simulink model "PV_MPPT"  (R2022b)
settings: Solver=VariableStepAuto  StartTime=0.0  StopTime=0.2  RelTol=1e-3
model workspace (MAT data in the model file):
  Tn = 298
undefined symbols (not defined in the file): sigbuilder_block
libraries: spsSeriesRLCBranchLib x4, spsCurrentMeasurementLib x1, spsGroundLib x1, spsIGBTLib x1, spsControlledCurrentSourceLib x1, spsPWMGeneratorDCDCLib x1, simulink x1, spsDiodeLib x1, spsVoltageMeasurementLib x1, spspowerguiLib x1
settings Model: Creator=Administrator  LastModifiedBy=58239
settings DebuggingCC: AlgebraicLoopMsg=none
settings ModelReferenceCC: EnableRefExpFcnMdlSchedulingChecks=on

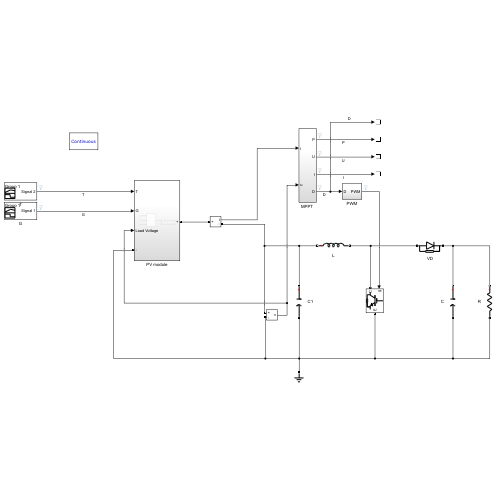
[thumbnail: Simulink's stored preview of the top-level diagram]
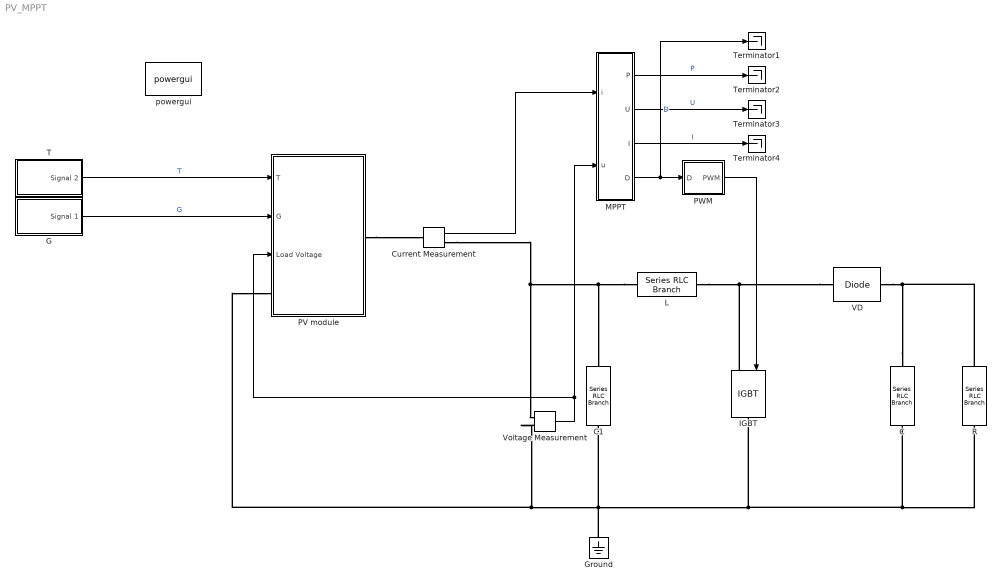
== system PV_MPPT ==
  C : spsSeriesRLCBranchLib/Series RLC Branch  LConnTagsString=__new0  RConnTagsString=__new0  BranchType=C  Resistance=0  Inductance=0  SetiL0=off  InitialCurrent=0  Capacitance=300e-6  Setx0=on  InitialVoltage=0  Measurements=None
  C1 : spsSeriesRLCBranchLib/Series RLC Branch  LConnTagsString=__new0  RConnTagsString=__new0  BranchType=C  Resistance=0  Inductance=0  SetiL0=off  InitialCurrent=0  Capacitance=300e-6  Setx0=off  InitialVoltage=0  Measurements=None
  Current Measurement : spsCurrentMeasurementLib/Current Measurement  PhasorSimulation=off  OutputType=Complex  PSBequivalent=0
  G : Subsystem  Tag=STV Subsys  LoadFcn=sigbuilder_block('load');  StartFcn=sigbuilder_block('start');  StopFcn=sigbuilder_block('stop');  ClipboardFcn=sigbuilder_block('clipboard');  mask(Sigbuilder block){tuvar=[0:10]}
      mask help: Sigbuilder GUI
      mask init:
      | if ~strcmp(get_param(bdroot(gcbh),'SimulationStatus'),'stopped') tuvar = sigbuilder_block('maskInit'); end
      settings: CopyFcn=sigbuilder_block('copy');  DeleteFcn=sigbuilder_block('delete');  ModelCloseFcn=sigbuilder_block('modelClose');  PreSaveFcn=sigbuilder_block('preSave');  PauseFcn=sigbuilder_block('pause')  ContinueFcn=sigbuilder_block('continue')  NameChangeFcn=sigbuilder_block('namechange');  OpenFcn=sigbuilder_block('open',[291 78 519 442.2 ]);  CloseFcn=sigbuilder_block('close');
      mask Display: plot(0, 0, 100, 100,[2, 2, 32, 32, 2], [68, 8, 8, 68, 68],[32, 2], [38, 38], [32, 19, 2],[53, 60, 44], [32, 17, 17, 2],[16, 16, 31, 31]);txt = getActiveGroup(gcbh);text(2, 100, txt,'verticalAlignment', 'top');
  Ground : spsGroundLib/Ground  LConnTagsString=a
  IGBT : spsIGBTLib/IGBT  Ron=0.00000001  Lon=0  Vf=1  Tf=1e-6  Tt=2e-6  IC=0  Rs=1e5  Cs=inf  Measurements=off
  L : spsSeriesRLCBranchLib/Series RLC Branch  LConnTagsString=__new0  RConnTagsString=__new0  BranchType=L  Resistance=0  Inductance=200e-6  SetiL0=off  InitialCurrent=1  Capacitance=inf  Setx0=off  InitialVoltage=0  Measurements=None
  "MPPT " : Subsystem
  PV module : Subsystem
  PWM : Subsystem
  R : spsSeriesRLCBranchLib/Series RLC Branch  LConnTagsString=__new0  RConnTagsString=__new0  BranchType=R  Resistance=30  Inductance=100e-6  SetiL0=off  InitialCurrent=0  Capacitance=inf  Setx0=off  InitialVoltage=0  Measurements=None
  T : Subsystem  Tag=STV Subsys  LoadFcn=sigbuilder_block('load');  StartFcn=sigbuilder_block('start');  StopFcn=sigbuilder_block('stop');  ClipboardFcn=sigbuilder_block('clipboard');  mask(Sigbuilder block){tuvar=[0:10]}
      mask help: Sigbuilder GUI
      mask init:
      | if ~strcmp(get_param(bdroot(gcbh),'SimulationStatus'),'stopped') tuvar = sigbuilder_block('maskInit'); end
      settings: CopyFcn=sigbuilder_block('copy');  DeleteFcn=sigbuilder_block('delete');  ModelCloseFcn=sigbuilder_block('modelClose');  PreSaveFcn=sigbuilder_block('preSave');  PauseFcn=sigbuilder_block('pause')  ContinueFcn=sigbuilder_block('continue')  NameChangeFcn=sigbuilder_block('namechange');  OpenFcn=sigbuilder_block('open',[317 199.5 519.5 400 ]);  CloseFcn=sigbuilder_block('close');
      mask Display: plot(0, 0, 100, 100,[2, 2, 32, 32, 2], [68, 8, 8, 68, 68],[32, 2], [38, 38], [32, 19, 2],[53, 60, 44], [32, 17, 17, 2],[16, 16, 31, 31]);txt = getActiveGroup(gcbh);text(2, 100, txt,'verticalAlignment', 'top');
  Terminator{1..4} (4 alike) : Terminator
  VD : spsDiodeLib/Diode  Ron=0.00000001  Lon=0  Vf=0.7  IC=0  UseSnubber=off  Rs=500  Cs=250e-9  Measurements=off
  Voltage Measurement : spsVoltageMeasurementLib/Voltage Measurement  PhasorSimulation=off  OutputType=Complex  PSBequivalent=0
  powergui : spspowerguiLib/powergui  Priority=1  SimulationMode=Continuous  SampleTime=50e-8  frequency=60  Iterations=50  frequencyindice=0  Pbase=100e6  ErrMax=1e-4  UnitsV=kV  UnitsW=MW  buscounter=0  FunctionMessages=off  echomessages=off  EnableUseOfTLC=off  CurrentSourceSwitches=off  DisableSnubberDevices=off  DisableRonSwitches=off  DisableVfSwitches=off  DisplayEquations=off  AutomaticDiscreteSolvers=off  SolverType=Tustin/Backward Euler (TBE)  Interpol=off  ExternalGateDelay=off  methode=off  Ts=100  x0status=blocks  SPID=off  SwTol=0  HookPort=off  NonlinearTolerance=1e-4  nMaxIteration=100  ContinueOnMaxIteration=off  RestoreLinks=warning  ResistiveCurrentMeasurement=off  Frange=[0:2:500]  Ylog=off  Xlog=on  ShowGrid=off  save=off  variable=ZData  structure=0  ZoomFFT=off  StartTime=0.0  cycles=1  DisplayStyle=1  fundamental=60  FreqAxis=off  MaxFrequency=1000  frequencyindicesteady=1  RmsSteady=1  display=off
  wires:
  "MPPT "/4(D) -> Terminator1/1, PWM/1(D)  "D"
  Current Measurement/1 -> "MPPT "/1(i)
  "MPPT "/2(U) -> Terminator3/1  "U"
  PWM/1(PWM) -> IGBT/1
  "MPPT "/1(P) -> Terminator2/1  "P"
  Voltage Measurement/1 -> PV module/3(Load Voltage), "MPPT "/2(u)
  "MPPT "/3(I) -> Terminator4/1  "I"
  T/1(Signal 2) -> PV module/1(T)  "T"
  G/1(Signal 1) -> PV module/2(G)  "G"
  connections:
  VD/LConn1 -- L/RConn1 -- IGBT/LConn1
  Voltage Measurement/LConn2 -- PV module/LConn1 -- Ground/LConn1 -- C1/RConn1 -- C/RConn1 -- R/RConn1 -- IGBT/RConn1
  C/LConn1 -- VD/RConn1 -- R/LConn1
  L/LConn1 -- Current Measurement/RConn1 -- Voltage Measurement/LConn1 -- C1/LConn1
  PV module/RConn1 -- Current Measurement/LConn1

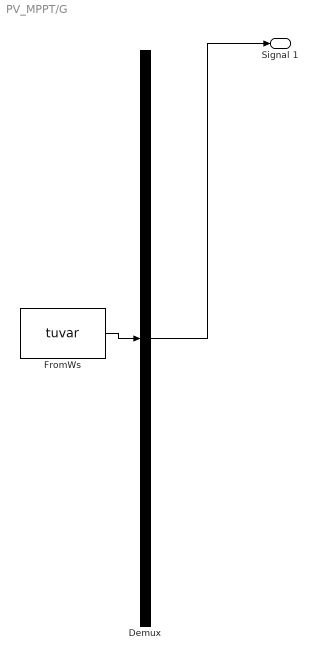
== system PV_MPPT/G ==
  Demux : Demux  Tag=STV Demux  Outputs=1
      settings: DisplayOption=none
  FromWs : FromWorkspace  Tag=STV FromWs  VariableName=tuvar  ZeroCross=off
      SigBuilderData=|
      | dataSet.timeRange = [0 0.16]
      | dataSet.name = 'Group 1'
      | sbobj.Groups.Name = 'Group 1'
      | sbobj.Groups.Signals.Name = 'Signal 1'
      | sbobj.Groups.Signals.XData = [0 0.0795 0.16]
      | sbobj.Groups.Signals.YData = [1000 1149.5 1001]
      | sbobj.Groups.TimeRange = [0 0.16]
  Signal 1 : Outport  Tag=STV Outport
  wires:
  FromWs/1 -> Demux/1
  Demux/1 -> Signal 1/1

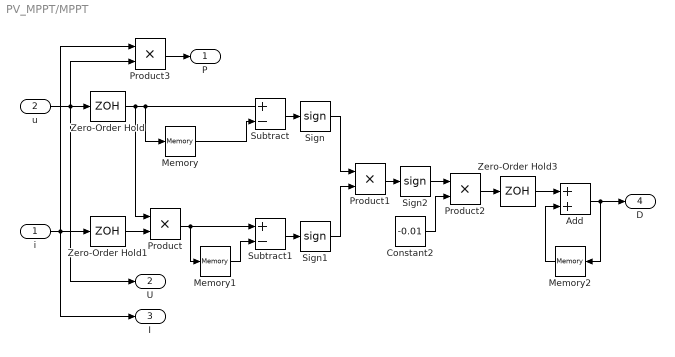
== system PV_MPPT/MPPT  ==
  i : Inport
  u : Inport  Port=2
  Add : Sum
  Constant2 : Constant  Value=-0.01
  Memory : Memory  InheritSampleTime=on
  Memory1 : Memory  InheritSampleTime=on
  Memory2 : Memory  InitialCondition=1  InheritSampleTime=on
  Product{,1..3} (4 alike) : Product  RndMeth=Zero
  Sign : Signum
  Sign1 : Signum
  Sign2 : Signum
  Subtract : Sum  Inputs=+-
  Subtract1 : Sum  Inputs=+-
  Zero-Order Hold : ZeroOrderHold  SampleTime=0.0005
  Zero-Order Hold1 : ZeroOrderHold  SampleTime=0.0005
  Zero-Order Hold3 : ZeroOrderHold  SampleTime=0.0005
  P : Outport
  U : Outport  Port=2
  I : Outport  Port=3
  D : Outport  Port=4
  wires:
  u/1 -> Zero-Order Hold/1, Product3/2, U/1
  i/1 -> Zero-Order Hold1/1, Product3/1, I/1
  Zero-Order Hold/1 -> Product/1, Subtract/1, Memory/1
  Memory/1 -> Subtract/2
  Zero-Order Hold1/1 -> Product/2
  Product/1 -> Subtract1/1, Memory1/1
  Memory1/1 -> Subtract1/2
  Subtract/1 -> Sign/1
  Subtract1/1 -> Sign1/1
  Sign/1 -> Product1/1
  Sign1/1 -> Product1/2
  Product1/1 -> Sign2/1
  Sign2/1 -> Product2/1
  Add/1 -> Memory2/1, D/1
  Memory2/1 -> Add/2
  Constant2/1 -> Product2/2
  Product3/1 -> P/1
  Product2/1 -> Zero-Order Hold3/1
  Zero-Order Hold3/1 -> Add/1

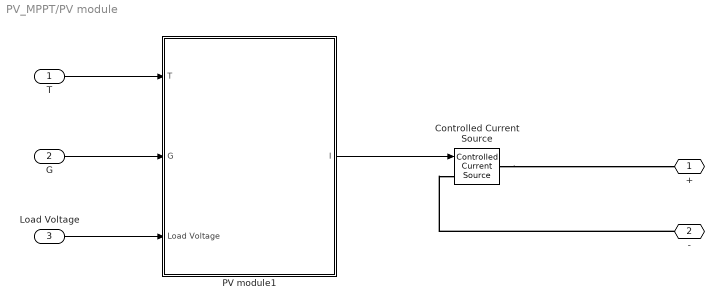
== system PV_MPPT/PV module ==
  T : Inport
  G : Inport  Port=2
  Load Voltage : Inport  Port=3
  Controlled Current Source : spsControlledCurrentSourceLib/Controlled Current Source  Initialize=on  Source_Type=AC  Amplitude=0  Phase=0  Frequency=0  Measurements=None
  PV module1 : Subsystem  mask{ki=0.0032, q=1.6e-19, K=1.38e-23, n=1.3, Eg0=1.1, Rs=0.221, Rsh=415.405, Tn=298, Voc=32.9, Isc=8.21, Ns=54}
      mask DialogControl DescGroupVar Prompt: PV Module
      mask DialogControl DescTextVar Prompt: 更改下列参数，以达到仿真效果。
      mask DialogControl ParameterGroupVar Prompt: 参数
  + : PMIOPort  Side=Right
  - : PMIOPort  Port=2  Side=Left
  wires:
  PV module1/1(I) -> Controlled Current Source/1
  Load Voltage/1 -> PV module1/3(Load Voltage)
  T/1 -> PV module1/1(T)
  G/1 -> PV module1/2(G)
  connections:
  -/RConn1 -- Controlled Current Source/LConn1
  Controlled Current Source/RConn1 -- +/RConn1

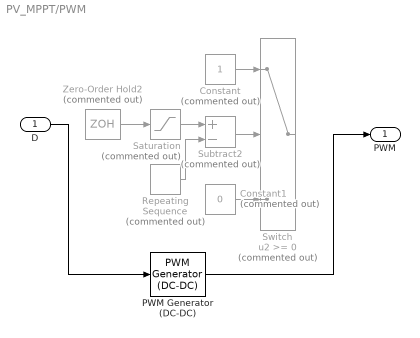
== system PV_MPPT/PWM ==
  D : Inport
  Constant : Constant  Commented=on
  Constant1 : Constant  Commented=on  Value=0
  PWM Generator (DC-DC) : spsPWMGeneratorDCDCLib/PWM Generator (DC-DC)  Fsw=5000  Ts=0
  Repeating Sequence : simulink/Sources/Repeating Sequence  Commented=on  rep_seq_t=[0 0.0001]  rep_seq_y=[0 1]
  Saturation : Saturate  Commented=on  UpperLimit=1  LowerLimit=0
  Subtract2 : Sum  Commented=on  Inputs=+-
  Switch : Switch  Commented=on  SaturateOnIntegerOverflow=off  InputSameDT=off
  Zero-Order Hold2 : ZeroOrderHold  Commented=on  SampleTime=0.0005
  PWM : Outport
  wires:
  Zero-Order Hold2/1 -> Saturation/1
  Constant1/1 -> Switch/3
  Constant/1 -> Switch/1
  Subtract2/1 -> Switch/2
  Repeating Sequence/1 -> Subtract2/2
  Saturation/1 -> Subtract2/1
  D/1 -> PWM Generator (DC-DC)/1
  PWM Generator (DC-DC)/1 -> PWM/1

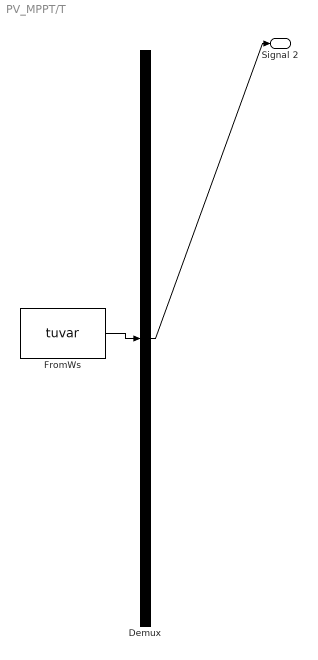
== system PV_MPPT/T ==
  Demux : Demux  Tag=STV Demux  Outputs=1
      settings: DisplayOption=none
  FromWs : FromWorkspace  Tag=STV FromWs  VariableName=tuvar  ZeroCross=off
      SigBuilderData=|
      | dataSet.timeRange = [0 0.16]
      | dataSet.name = 'Group 1'
      | sbobj.Groups.Name = 'Group 1'
      | sbobj.Groups.Signals.Name = 'Signal 2'
      | sbobj.Groups.Signals.XData = [0 0.0805 0.16]
      | sbobj.Groups.Signals.YData = [25 20.1 25.01]
      | sbobj.Groups.TimeRange = [0 0.16]
  Signal 2 : Outport  Tag=STV Outport
  wires:
  FromWs/1 -> Demux/1
  Demux/1 -> Signal 2/1

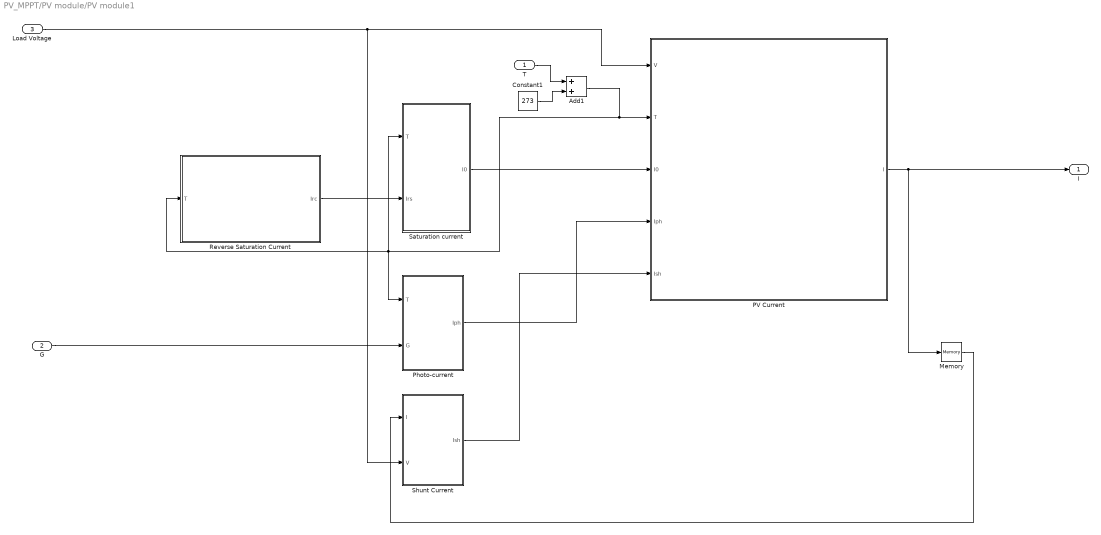
== system PV_MPPT/PV module/PV module1 ==
  T : Inport
  G : Inport  Port=2
  Load Voltage : Inport  Port=3
  Add1 : Sum
  Constant1 : Constant  Value=273
  Memory : Memory
  PV Current : Subsystem
  Photo-current : Subsystem
  Reverse Saturation Current : Subsystem
  Saturation current : Subsystem
  Shunt Current : Subsystem
  I : Outport
  wires:
  Shunt Current/1(Ish) -> PV Current/5(Ish)
  Load Voltage/1 -> Shunt Current/2(V), PV Current/1(V)
  Saturation current/1(I0) -> PV Current/3(I0)
  PV Current/1(I) -> Memory/1, I/1
  G/1 -> Photo-current/2(G)
  Reverse Saturation Current/1(Irc) -> Saturation current/2(Irs)
  Add1/1 -> Reverse Saturation Current/1(T), Saturation current/1(T), Photo-current/1(T), PV Current/2(T)
  Photo-current/1(Iph) -> PV Current/4(Iph)
  T/1 -> Add1/1
  Constant1/1 -> Add1/2
  Memory/1 -> Shunt Current/1(I)

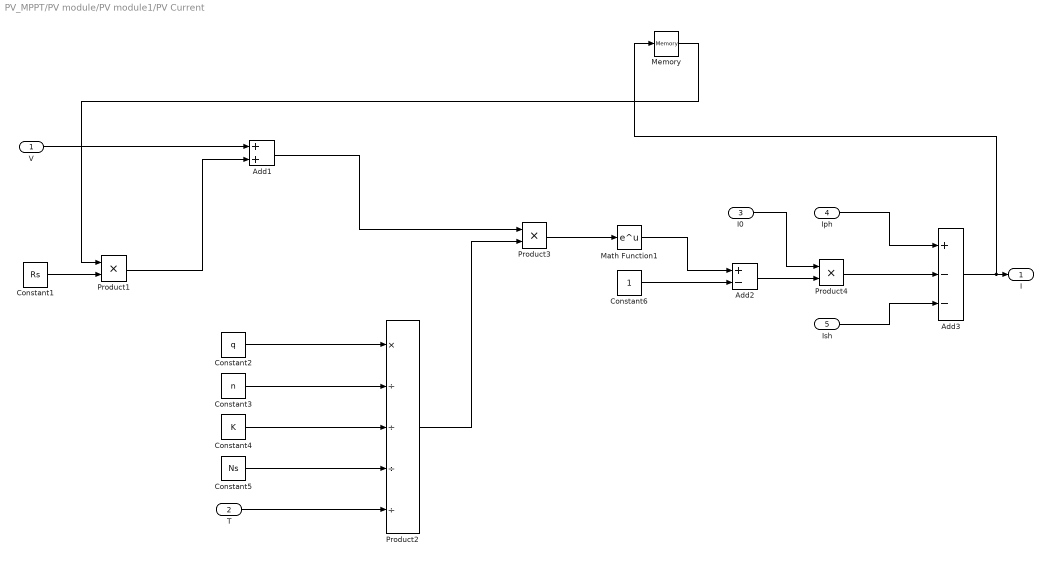
== system PV_MPPT/PV module/PV module1/PV Current ==
  V : Inport
  T : Inport  Port=2
  I0 : Inport  Port=3
  Iph : Inport  Port=4
  Ish : Inport  Port=5
  Add1 : Sum
  Add2 : Sum  Inputs=+-
  Add3 : Sum  Inputs=+--
  Constant1 : Constant  Value=Rs
  Constant2 : Constant  Value=q
  Constant3 : Constant  Value=n
  Constant4 : Constant  Value=K
  Constant5 : Constant  Value=Ns
  Constant6 : Constant
  Math Function1 : Math
  Memory : Memory
  Product1 : Product
  Product2 : Product  Inputs=*////
  Product3 : Product
  Product4 : Product
  I : Outport
  wires:
  Add1/1 -> Product3/1
  V/1 -> Add1/1
  Add3/1 -> Memory/1, I/1
  Add2/1 -> Product4/2
  Product3/1 -> Math Function1/1
  Iph/1 -> Add3/1
  Product1/1 -> Add1/2
  Constant1/1 -> Product1/2
  Math Function1/1 -> Add2/1
  T/1 -> Product2/5
  Product2/1 -> Product3/2
  Constant5/1 -> Product2/4
  Constant3/1 -> Product2/2
  Constant4/1 -> Product2/3
  Constant2/1 -> Product2/1
  Product4/1 -> Add3/2
  I0/1 -> Product4/1
  Constant6/1 -> Add2/2
  Ish/1 -> Add3/3
  Memory/1 -> Product1/1

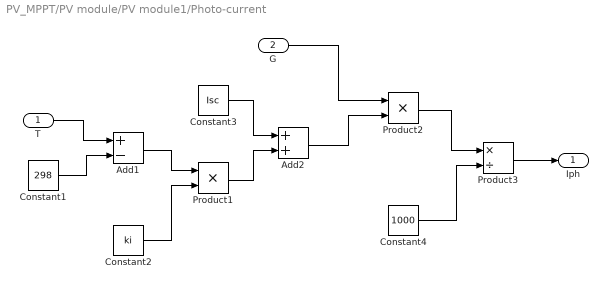
== system PV_MPPT/PV module/PV module1/Photo-current ==
  T : Inport
  G : Inport  Port=2
  Add1 : Sum  Inputs=+-
  Add2 : Sum
  Constant1 : Constant  Value=298
  Constant2 : Constant  Value=ki
  Constant3 : Constant  Value=Isc
  Constant4 : Constant  Value=1000
  Product1 : Product
  Product2 : Product
  Product3 : Product  Inputs=*/
  Iph : Outport
  wires:
  T/1 -> Add1/1
  G/1 -> Product2/1
  Product1/1 -> Add2/2
  Constant4/1 -> Product3/2
  Constant2/1 -> Product1/2
  Product3/1 -> Iph/1
  Constant3/1 -> Add2/1
  Add1/1 -> Product1/1
  Constant1/1 -> Add1/2
  Add2/1 -> Product2/2
  Product2/1 -> Product3/1

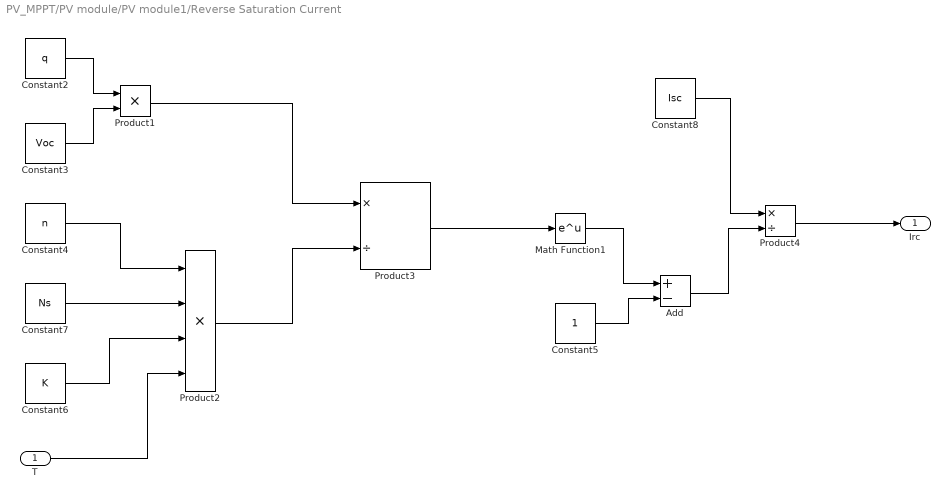
== system PV_MPPT/PV module/PV module1/Reverse Saturation Current ==
  T : Inport
  Add : Sum  Inputs=+-
  Constant2 : Constant  Value=q  SampleTime=-1
  Constant3 : Constant  Value=Voc  SampleTime=-1
  Constant4 : Constant  Value=n  SampleTime=-1
  Constant5 : Constant  VectorParams1D=off  SampleTime=-1
  Constant6 : Constant  Value=K  SampleTime=-1
  Constant7 : Constant  Value=Ns  SampleTime=-1
  Constant8 : Constant  Value=Isc  SampleTime=-1
  Math Function1 : Math
  Product1 : Product
  Product2 : Product  Inputs=4
  Product3 : Product  Inputs=*/
  Product4 : Product  Inputs=*/
  Irc : Outport
  wires:
  Product4/1 -> Irc/1
  Product2/1 -> Product3/2
  T/1 -> Product2/4
  Constant5/1 -> Add/2
  Constant2/1 -> Product1/1
  Product3/1 -> Math Function1/1
  Add/1 -> Product4/2
  Constant8/1 -> Product4/1
  Constant3/1 -> Product1/2
  Constant7/1 -> Product2/2
  Constant4/1 -> Product2/1
  Constant6/1 -> Product2/3
  Math Function1/1 -> Add/1
  Product1/1 -> Product3/1

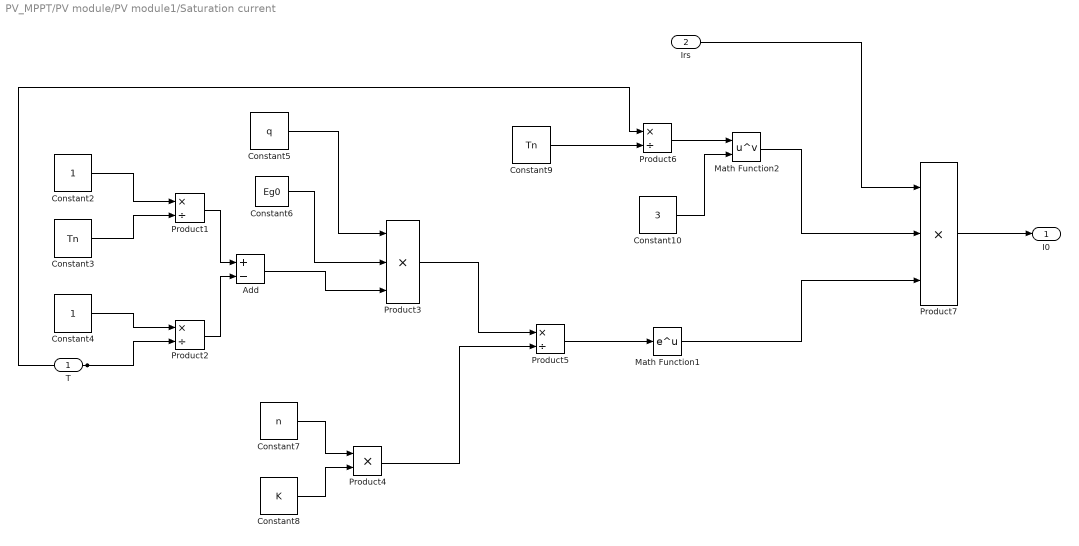
== system PV_MPPT/PV module/PV module1/Saturation current ==
  T : Inport
  Irs : Inport  Port=2
  Add : Sum  Inputs=+-
  Constant10 : Constant  Value=3  VectorParams1D=off  SampleTime=-1
  Constant2 : Constant  VectorParams1D=off  SampleTime=-1
  Constant3 : Constant  Value=Tn  SampleTime=-1
  Constant4 : Constant  VectorParams1D=off  SampleTime=-1
  Constant5 : Constant  Value=q  SampleTime=-1
  Constant6 : Constant  Value=Eg0  SampleTime=-1
  Constant7 : Constant  Value=n  SampleTime=-1
  Constant8 : Constant  Value=K  SampleTime=-1
  Constant9 : Constant  Value=Tn  SampleTime=-1
  Math Function1 : Math
  Math Function2 : Math  Operator=pow
  Product{1..2,5..6} (4 alike) : Product  Inputs=*/
  Product3 : Product  Inputs=3
  Product4 : Product
  Product7 : Product  Inputs=3
  I0 : Outport
  wires:
  T/1 -> Product2/2, Product6/1
  Constant7/1 -> Product4/1
  Product6/1 -> Math Function2/1
  Math Function1/1 -> Product7/3
  Constant2/1 -> Product1/1
  Constant4/1 -> Product2/1
  Product3/1 -> Product5/1
  Add/1 -> Product3/3
  Irs/1 -> Product7/1
  Constant3/1 -> Product1/2
  Math Function2/1 -> Product7/2
  Constant10/1 -> Math Function2/2
  Product1/1 -> Add/1
  Constant8/1 -> Product4/2
  Constant9/1 -> Product6/2
  Product4/1 -> Product5/2
  Constant6/1 -> Product3/2
  Product7/1 -> I0/1
  Product5/1 -> Math Function1/1
  Constant5/1 -> Product3/1
  Product2/1 -> Add/2

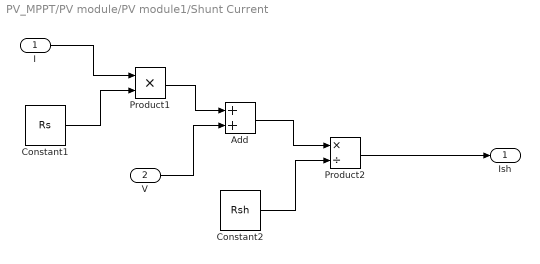
== system PV_MPPT/PV module/PV module1/Shunt Current ==
  I : Inport
  V : Inport  Port=2
  Add : Sum
  Constant1 : Constant  Value=Rs  SampleTime=-1
  Constant2 : Constant  Value=Rsh  SampleTime=-1
  Product1 : Product
  Product2 : Product  Inputs=*/
  Ish : Outport
  wires:
  I/1 -> Product1/1
  Constant1/1 -> Product1/2
  Product2/1 -> Ish/1
  Constant2/1 -> Product2/2
  V/1 -> Add/2
  Add/1 -> Product2/1
  Product1/1 -> Add/1
